simulink model "gm_EncoderRead"  (R2014b)
settings: Solver=FixedStepDiscrete  SolverMode=SingleTasking  StartTime=0.0  StopTime=50  FixedStep=1  RelTol=1e-3
settings Model: FPTRunName=FPA_Reference  Creator=variable  LastModifiedBy=dlwalter
settings DataIOCC: LimitDataPoints=off  SaveOutput=off  DSMLogging=off  SaveTime=off
settings OptimizationCC: BlockReduction=off  ConditionallyExecuteInputs=off  InlineParams=on
settings DebuggingCC: SignalRangeChecking=warning  AlgebraicLoopMsg=error  InheritedTsInSrcMsg=none  SingleTaskRateTransMsg=error  ParameterDowncastMsg=warning  ParameterOverflowMsg=warning  LoggingUnavailableSignals=none
settings HardwareCC: ProdHWDeviceType=ASIC/FPGA->ASIC/FPGA  TargetLongLongMode=on  TargetIntDivRoundTo=Zero  TargetEndianess=LittleEndian  TargetHWDeviceType=MATLAB Host  ProdEqTarget=off

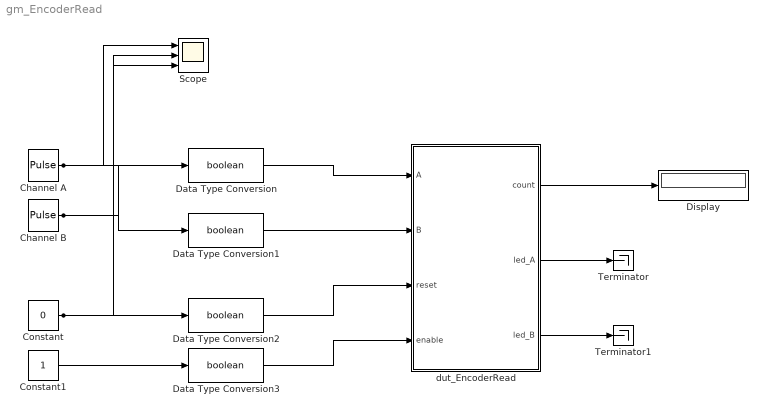
== system gm_EncoderRead ==
  Channel A : DiscretePulseGenerator  PulseType=Time based  Period=4  PulseWidth=50  PhaseDelay=1
  Channel B : DiscretePulseGenerator  PulseType=Time based  Period=4  PulseWidth=50
  Constant : Constant  Value=0  SampleTime=-1
  Constant1 : Constant  SampleTime=-1
  Data Type Conversion{,1..3} (4 alike) : DataTypeConversion  OutDataTypeStr=boolean
  Display : Display
  Scope : Scope  NumInputPorts=3
      settings: YMin=-5~-5~-5  YMax=5~5~5
  Terminator : Terminator
  Terminator1 : Terminator
  dut_EncoderRead : Subsystem  TreatAsAtomicUnit=on  MinMaxOverflowLogging=MinMaxAndOverflow
  wires:
  dut_EncoderRead/3(led_B) -> Terminator1/1
  dut_EncoderRead/2(led_A) -> Terminator/1
  dut_EncoderRead/1(count) -> Display/1
  Data Type Conversion3/1 -> dut_EncoderRead/4(enable)
  Data Type Conversion2/1 -> dut_EncoderRead/3(reset)
  Data Type Conversion1/1 -> dut_EncoderRead/2(B)
  Data Type Conversion/1 -> dut_EncoderRead/1(A)
  Constant1/1 -> Data Type Conversion3/1
  Channel B/1 -> Data Type Conversion/1, Scope/2
  Channel A/1 -> Scope/1, Data Type Conversion1/1
  Constant/1 -> Data Type Conversion2/1, Scope/3

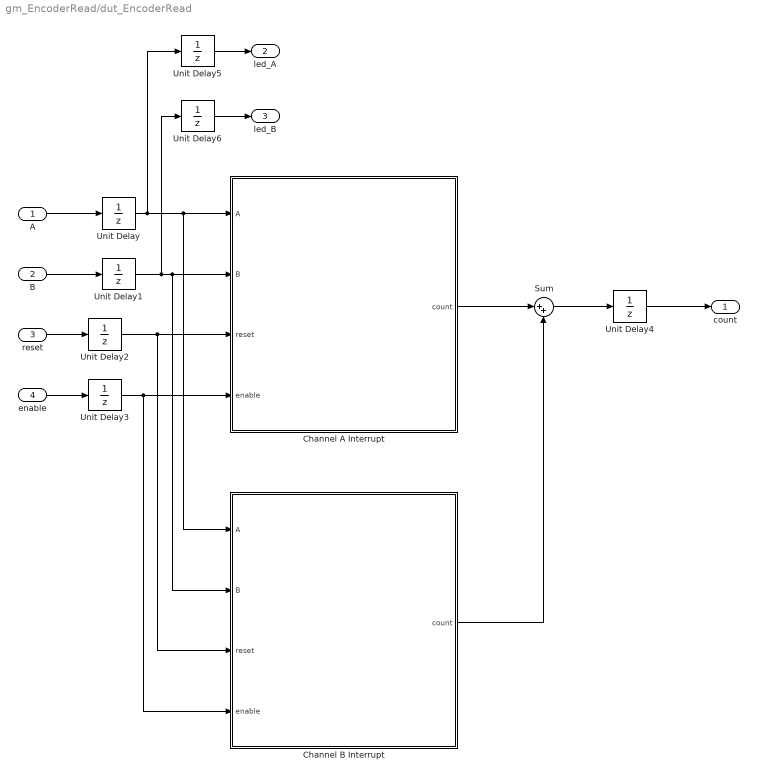
== system gm_EncoderRead/dut_EncoderRead ==
  A : Inport
  B : Inport  Port=2
  reset : Inport  Port=3
  enable : Inport  Port=4
  Channel A Interrupt : Stateflow chart  TreatAsAtomicUnit=on
  Channel B Interrupt : Stateflow chart  TreatAsAtomicUnit=on
  Sum : Sum  Inputs=|++  AccumDataTypeStr=int32
  Unit Delay{,1..6} (7 alike) : UnitDelay  SampleTime=-1
  count : Outport
  led_A : Outport  Port=2
  led_B : Outport  Port=3
  wires:
  Unit Delay6/1 -> led_B/1
  Unit Delay5/1 -> led_A/1
  Unit Delay4/1 -> count/1
  Unit Delay3/1 -> Channel A Interrupt/4(enable), Channel B Interrupt/4(enable)
  Unit Delay2/1 -> Channel A Interrupt/3(reset), Channel B Interrupt/3(reset)
  Unit Delay1/1 -> Channel A Interrupt/2(B), Channel B Interrupt/2(B), Unit Delay6/1
  Unit Delay/1 -> Channel A Interrupt/1(A), Channel B Interrupt/1(A), Unit Delay5/1
  Channel B Interrupt/1(count) -> Sum/2
  Sum/1 -> Unit Delay4/1
  enable/1 -> Unit Delay3/1
  reset/1 -> Unit Delay2/1
  B/1 -> Unit Delay1/1
  A/1 -> Unit Delay/1
  Channel A Interrupt/1(count) -> Sum/1

== stateflow chart gm_EncoderRead/dut_EncoderRead/Channel B Interrupt ==
  settings: executeAtInitialization=1
  state I4
  state I1
  state I2
  state I3
  (default) -> I4
  I3 -> I4
  I4 -> I1 : [enable == true]{count = int32(0); reset_val = reset;}
  (junction 22) -> I2 [order 1] : [A==B]{count = count - 1;}
  I1 -> (junction 22) [order 2] : [B==true]
  (junction 22) -> I2 [order 2] : [A~=B]{count = count + 1;}
  I2 -> I2 [order 3] : [reset ~= reset_val]
      | {count = int32(0); reset_val = reset;}
  I1 -> I1 [order 3] : [reset ~= reset_val]
      | {count = int32(0);reset_val = reset;}
  (junction 23) -> I1 [order 2] : [A ~= B]{count = count + 1;}
  I1 -> I3 [order 1] : [enable == false]
  (junction 23) -> I1 [order 1] : [A == B]{count = count - 1;}
  I2 -> I3 [order 2] : [enable == false]
  I2 -> (junction 23) [order 1] : [B == false]
  data: A input boolean; B input boolean; count output int32; reset input boolean; reset_val local boolean; enable input boolean

== stateflow chart gm_EncoderRead/dut_EncoderRead/Channel A Interrupt ==
  settings: executeAtInitialization=1
  state I4
  state I1
  state I2
  state I3
  (default) -> I4
  I3 -> I4
  I4 -> I1 : [enable == true]{count = int32(0); reset_val = reset;}
  (junction 22) -> I2 [order 1] : [A==B]{count = count + 1;}
  I1 -> (junction 22) [order 1] : [A==true]
  (junction 22) -> I2 [order 2] : [A~=B]{count = count - 1;}
  I2 -> I2 [order 3] : [reset ~= reset_val]
      | {count = int32(0); reset_val = reset;}
  I1 -> I1 [order 3] : [reset ~= reset_val]
      | {count =int32(0);reset_val = reset;}
  (junction 23) -> I1 [order 2] : [A ~= B]{count = count - 1;}
  I1 -> I3 [order 2] : [enable == false]
  (junction 23) -> I1 [order 1] : [A == B]{count = count + 1;}
  I2 -> I3 [order 2] : [enable == false]
  I2 -> (junction 23) [order 1] : [A == false]
  data: A input boolean; B input boolean; count output int32; reset input boolean; reset_val local boolean; enable input boolean
